simulink model "KITTDynamicsFinal"  (R2016b)
settings: Solver=VariableStepAuto  StartTime=0.0  StopTime=8  MaxStep=0.01  RelTol=1e-3
values from neighbouring files (symbols this model uses):
  b = 0.0015    [KITTParameters.m]
  c = 0.02    [KITTParameters.m]
  F_a_max = 80    [KITTParameters.m]
  F_b_max = 120    [KITTParameters.m]
  m = 13    [KITTParameters.m]
settings Model: Creator=sumeetsharma  LastModifiedBy=Sieger

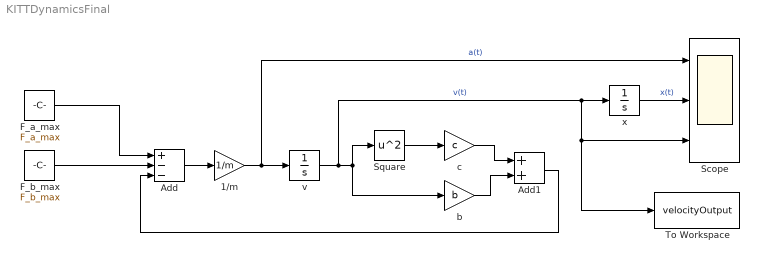
== system KITTDynamicsFinal ==
  1/m : Gain  Gain=1/m
  Add : Sum  Inputs=+--
  Add1 : Sum
  F_a_max : Constant  Value=F_a_max
  "F_b_max " : Constant  Value=F_b_max
  Scope : Scope  NumInputPorts=3
  Square : Math  Operator=square  SaturateOnIntegerOverflow=on
  To Workspace : ToWorkspace  VariableName=velocityOutput  SaveFormat=Structure With Time  SampleTime=-1
  b : Gain  Gain=b
  c : Gain  InitFcn=run KITTParameters.m  Gain=c
  v : Integrator  InitialCondition=1
  "x " : Integrator
  wires:
  F_a_max/1 -> Add/1
  "F_b_max "/1 -> Add/2
  Add/1 -> 1/m/1
  1/m/1 -> Scope/1, v/1  "a(t)"
  v/1 -> Scope/3, To Workspace/1, "x "/1, b/1, Square/1  "v(t)"
  Square/1 -> c/1
  c/1 -> Add1/1
  b/1 -> Add1/2
  Add1/1 -> Add/3
  "x "/1 -> Scope/2  "x(t)"
